simulink model "untitled"  (Simulink 7.9)
settings: Solver=ode45  StartTime=0.0  StopTime=10.0  RelTol=1e-3
settings Model: Creator=thinkpad  LastModifiedBy=thinkpad

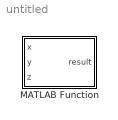
== system untitled ==
  MATLAB Function : MATLAB Function  TreatAsAtomicUnit=on

== matlab function MATLAB Function ==
  data: x input double; y input double; z input double; result output double
function result = fcn(x,y,z)
%#codegen

result = x + sin(y) + fft2(z);
